simulink model "motorStyrning"  (R2020b)
settings: Solver=VariableStepAuto  StartTime=0.0  StopTime=0.1  RelTol=1e-3
model workspace (MAT data in the model file):
  intervall = 300
  intervall2 = 1
  intervall3 = 1
  timeTTT : Simulink.Signal (value not decoded)
libraries: fl_lib x116, ee_lib x24, nesl_utility x23
(part 2 of 2)

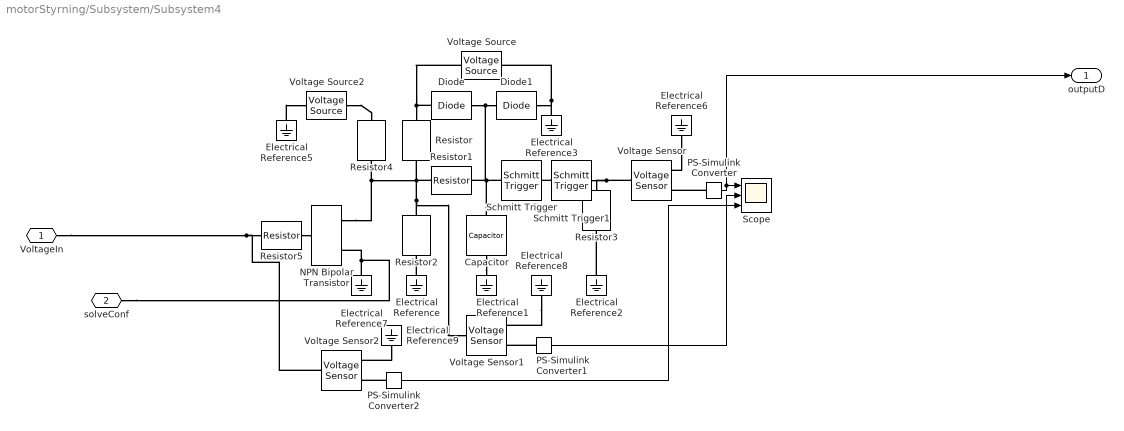
== system motorStyrning/Subsystem/Subsystem4 ==
  Capacitor : fl_lib/Electrical/Electrical Elements/Capacitor  c=100 nF  r=1e-6 Ohm  g=0 1/Ohm  i_specify=off  i_priority=None  i=0 A  i_nominal_specify=off  i_nominal_unit=A  i_nominal_value=1  v_specify=off  v_priority=None  v=0 V  v_nominal_specify=off  v_nominal_unit=V  v_nominal_value=1  vc_specify=off  vc_priority=High  vc=0 V  vc_nominal_specify=off  vc_nominal_unit=V  vc_nominal_value=1
  Diode : ee_lib/Semiconductors & Converters/Diode  ModelType=ee.enum.diode.modelType.pwl  IfMat=[.07, .12, .19, 1.75, 4.24, 7.32, 11.2; .16, .3, .72, 2.14, 4.02, 6.35, 9.12] A  TjVec=[25, 125] degC  VfVec=[.5, .7, .9, 1.3, 1.7, 2.1, 2.5] V  Vf=0.6 V  Ron=0.3 Ohm  Goff=1e-8 S  prmExp=ee.enum.diode.expParam.useTwo  I12=[.0137, .545] A  V12=[.6, .7] V  IS=1e-12 A  ec=1  I1=0.0137 A  V1=0.6 V  RS=0 Ohm  Tmeas=25 degC  N_series=1  N_parallel=1  Rz=0.3 Ohm  BV=inf V  C_param=ee.enum.diode.capParam.fixed  CJ=5 pF  CJ0=5 pF  VJ=1 V  Mgrad=0.5  Vvec=[.1, 10, 100] V  Cvec=[3.5, 1, .4] pF  FC=0.5  Q_param=ee.enum.diode.recoveryParam.off  iRM=-7.15 A  iF=4 A  didt=-750 A/us  trr_factor=3  trr=115 ns  Qrr=1500 s*uA  TT=50 ns  tau=100 ns  T_param=ee.enum.diode.temperatureParam.off  IS_T2=1.25e-7 A  I1_T2=0.245 A  V1_T2=0.5 V  Tmeas2=125 degC  EG_param=ee.enum.diode.egapParam.material_si  EG=1.11 eV  XTI_param=ee.enum.diode.xtiParam.pn  XTI=3  dBVdT=0 V/K  Tdevice=25 degC  i_specify=off  i_priority=None  i=0 A  i_nominal_specify=off  i_nominal_unit=A  i_nominal_value=1  v_specify=off  v_priority=None  v=0 V  v_nominal_specify=off  v_nominal_unit=V  v_nominal_value=1  i_capacitor_specify=off  i_capacitor_priority=None  i_capacitor=0 A  i_capacitor_nominal_specify=off  i_capacitor_nominal_unit=A  i_capacitor_nominal_value=1  v_capacitor_specify=off  v_capacitor_priority=None  v_capacitor=0 V  v_capacitor_nominal_specify=off  v_capacitor_nominal_unit=V  v_capacitor_nominal_value=1  power_dissipated_specify=off  power_dissipated_priority=None  power_dissipated=0 W  power_dissipated_nominal_specify=off  power_dissipated_nominal_unit=W  power_dissipated_nominal_value=1  thermal_network_parameterization=ee.enum.thermalNetworkTopology.cauer  Rth=[0, 10] K/W  Rth_Foster=[4, 6] K/W  thermal_mass_parameterization=ee.enum.thermalNetwork.timeconstant  thermal_mass=[0, 1] J/K  thermal_mass_Foster=[1.5, 3] J/K  thermal_time_constant=[0, 10] s  thermal_time_constant_Foster=[6, 18] s  thermal_mass_initial_temperatures=[25, 25] degC
  Diode1 : ee_lib/Semiconductors & Converters/Diode  ModelType=ee.enum.diode.modelType.pwl  IfMat=[.07, .12, .19, 1.75, 4.24, 7.32, 11.2; .16, .3, .72, 2.14, 4.02, 6.35, 9.12] A  TjVec=[25, 125] degC  VfVec=[.5, .7, .9, 1.3, 1.7, 2.1, 2.5] V  Vf=0.6 V  Ron=0.3 Ohm  Goff=1e-8 S  prmExp=ee.enum.diode.expParam.useTwo  I12=[.0137, .545] A  V12=[.6, .7] V  IS=1e-12 A  ec=1  I1=0.0137 A  V1=0.6 V  RS=0 Ohm  Tmeas=25 degC  N_series=1  N_parallel=1  Rz=0.3 Ohm  BV=inf V  C_param=ee.enum.diode.capParam.fixed  CJ=5 pF  CJ0=5 pF  VJ=1 V  Mgrad=0.5  Vvec=[.1, 10, 100] V  Cvec=[3.5, 1, .4] pF  FC=0.5  Q_param=ee.enum.diode.recoveryParam.off  iRM=-7.15 A  iF=4 A  didt=-750 A/us  trr_factor=3  trr=115 ns  Qrr=1500 s*uA  TT=50 ns  tau=100 ns  T_param=ee.enum.diode.temperatureParam.off  IS_T2=1.25e-7 A  I1_T2=0.245 A  V1_T2=0.5 V  Tmeas2=125 degC  EG_param=ee.enum.diode.egapParam.material_si  EG=1.11 eV  XTI_param=ee.enum.diode.xtiParam.pn  XTI=3  dBVdT=0 V/K  Tdevice=25 degC  i_specify=off  i_priority=None  i=0 A  i_nominal_specify=off  i_nominal_unit=A  i_nominal_value=1  v_specify=off  v_priority=None  v=0 V  v_nominal_specify=off  v_nominal_unit=V  v_nominal_value=1  i_capacitor_specify=off  i_capacitor_priority=None  i_capacitor=0 A  i_capacitor_nominal_specify=off  i_capacitor_nominal_unit=A  i_capacitor_nominal_value=1  v_capacitor_specify=off  v_capacitor_priority=None  v_capacitor=0 V  v_capacitor_nominal_specify=off  v_capacitor_nominal_unit=V  v_capacitor_nominal_value=1  power_dissipated_specify=off  power_dissipated_priority=None  power_dissipated=0 W  power_dissipated_nominal_specify=off  power_dissipated_nominal_unit=W  power_dissipated_nominal_value=1  thermal_network_parameterization=ee.enum.thermalNetworkTopology.cauer  Rth=[0, 10] K/W  Rth_Foster=[4, 6] K/W  thermal_mass_parameterization=ee.enum.thermalNetwork.timeconstant  thermal_mass=[0, 1] J/K  thermal_mass_Foster=[1.5, 3] J/K  thermal_time_constant=[0, 10] s  thermal_time_constant_Foster=[6, 18] s  thermal_mass_initial_temperatures=[25, 25] degC
  Electrical Reference{,1..3,5..9} (9 alike) : fl_lib/Electrical/Electrical Elements/Electrical Reference
  NPN Bipolar Transistor : ee_lib/Semiconductors & Converters/NPN Bipolar Transistor  parameterization=1  prmDatasheet=1  prmEquCoeff=1  BF=100  IS=1e-14 A  VAF=200 V  hfe=100  hoe=50e-6 1/Ohm  Ic_h=1 mA  Vce_h=5 V  V1=0.55 V  I1=0.5 mA  BR=1  Tmeas=25 degC  RC=0.01 Ohm  RE=1e-4 Ohm  RB=1 Ohm  C_BC=5 pF  C_BE=5 pF  TF=0 us  TR=0 us  hfe_T2=125  XTB=0  V1_T2=0.45 V  I1_T2=0.5 mA  Tmeas2=125 degC  EG=1.11 eV  XTI=3  ec=1  TdeviceDatasheet=25 degC  TdeviceEquCoeff=25 degC  thermal_network_parameterization=ee.enum.thermalNetworkTopology.cauer  Rth=[0, 10] K/W  Rth_Foster=[4, 6] K/W  thermal_mass_parameterization=ee.enum.thermalNetwork.timeconstant  thermal_mass=[0, 1] J/K  thermal_mass_Foster=[1.5, 3] J/K  thermal_time_constant=[0, 10] s  thermal_time_constant_Foster=[6, 18] s  thermal_mass_initial_temperatures=[25, 25] degC
  PS-Simulink Converter : nesl_utility/PS-Simulink Converter  PhysicalDomain=network_engine_domain  SubClassName=ps_output  LeftPortType=input  RightPortType=output  PseudoPeriodic=off  Frequencies=[]  Unit=inherit  AffineConversion=off
  PS-Simulink Converter1 : nesl_utility/PS-Simulink Converter  PhysicalDomain=network_engine_domain  SubClassName=ps_output  LeftPortType=input  RightPortType=output  PseudoPeriodic=off  Frequencies=[]  Unit=inherit  AffineConversion=off
  PS-Simulink Converter2 : nesl_utility/PS-Simulink Converter  PhysicalDomain=network_engine_domain  SubClassName=ps_output  LeftPortType=input  RightPortType=output  PseudoPeriodic=off  Frequencies=[]  Unit=inherit  AffineConversion=off
  Resistor : fl_lib/Electrical/Electrical Elements/Resistor  R=1 kOhm  i_specify=off  i_priority=None  i=0 A  i_nominal_specify=off  i_nominal_unit=A  i_nominal_value=1  v_specify=off  v_priority=None  v=0 V  v_nominal_specify=off  v_nominal_unit=V  v_nominal_value=1
  Resistor1 : fl_lib/Electrical/Electrical Elements/Resistor  R=1 kOhm  i_specify=off  i_priority=None  i=0 A  i_nominal_specify=off  i_nominal_unit=A  i_nominal_value=1  v_specify=off  v_priority=None  v=0 V  v_nominal_specify=off  v_nominal_unit=V  v_nominal_value=1
  Resistor2 : fl_lib/Electrical/Electrical Elements/Resistor  R=50 kOhm  i_specify=off  i_priority=None  i=0 A  i_nominal_specify=off  i_nominal_unit=A  i_nominal_value=1  v_specify=off  v_priority=None  v=0 V  v_nominal_specify=off  v_nominal_unit=V  v_nominal_value=1
  Resistor3 : fl_lib/Electrical/Electrical Elements/Resistor  R=10 kOhm  i_specify=off  i_priority=None  i=0 A  i_nominal_specify=off  i_nominal_unit=A  i_nominal_value=1  v_specify=off  v_priority=None  v=0 V  v_nominal_specify=off  v_nominal_unit=V  v_nominal_value=1
  Resistor4 : fl_lib/Electrical/Electrical Elements/Resistor  R=10 kOhm  i_specify=off  i_priority=None  i=0 A  i_nominal_specify=off  i_nominal_unit=A  i_nominal_value=1  v_specify=off  v_priority=None  v=0 V  v_nominal_specify=off  v_nominal_unit=V  v_nominal_value=1
  Resistor5 : fl_lib/Electrical/Electrical Elements/Resistor  R=1 kOhm  i_specify=off  i_priority=None  i=0 A  i_nominal_specify=off  i_nominal_unit=A  i_nominal_value=1  v_specify=off  v_priority=None  v=0 V  v_nominal_specify=off  v_nominal_unit=V  v_nominal_value=1
  Schmitt Trigger : ee_lib/Integrated Circuits/Logic/Schmitt Trigger  V_IL=2 V  V_IH=3 V  C_IN=5 pF  output_type=1  V_OL=0 V  V_OH=5 V  V_CC=5 V  V_meas=5 V  R_OUT=25 Ohm  R_OH=[25, 250] Ohm  I_OH=63 mA  R_OL=[30, 800] Ohm  I_OL=-45 mA  Delay=25 ns  Ron=5 Ohm  Vf=0.6 V  output_state=1
      settings: SourceProductBaseCode=PS  InternalSimscapePortConfiguration="{\"Bottom\":[],\"Left\":[{\"id\":\"A\",\"label\":\"\",\"type\":\"foundation.electrical.electrical\"}],\"Right\":[{\"id\":\"J\",\"label\":\"\",\"type\":\"foundation.electrical.electrical\"}],\"Top\":[]}"
  Schmitt Trigger1 : ee_lib/Integrated Circuits/Logic/Schmitt Trigger  V_IL=2 V  V_IH=3 V  C_IN=5 pF  output_type=1  V_OL=0 V  V_OH=5 V  V_CC=5 V  V_meas=5 V  R_OUT=25 Ohm  R_OH=[25, 250] Ohm  I_OH=63 mA  R_OL=[30, 800] Ohm  I_OL=-45 mA  Delay=25 ns  Ron=5 Ohm  Vf=0.6 V  output_state=1
      settings: SourceProductBaseCode=PS  InternalSimscapePortConfiguration="{\"Bottom\":[],\"Left\":[{\"id\":\"A\",\"label\":\"\",\"type\":\"foundation.electrical.electrical\"}],\"Right\":[{\"id\":\"J\",\"label\":\"\",\"type\":\"foundation.electrical.electrical\"}],\"Top\":[]}"
  Scope : Scope  NumInputPorts=3
  Voltage Sensor : fl_lib/Electrical/Electrical Sensors/Voltage Sensor
  Voltage Sensor1 : fl_lib/Electrical/Electrical Sensors/Voltage Sensor
  Voltage Sensor2 : fl_lib/Electrical/Electrical Sensors/Voltage Sensor
  Voltage Source : ee_lib/Sources/Voltage Source  dc_voltage=5 V  ac_voltage=0 V  ac_shift=0 rad  ac_frequency=60 Hz  noise_mode=0  PSD=0 V^2/Hz  repeatability=1  auto_seed=4112460543  user_seed=0  sample_time=1e-3 s  i_specify=off  i_priority=None  i=0 A  i_nominal_specify=off  i_nominal_unit=A  i_nominal_value=1  v_specify=off  v_priority=None  v=0 V  v_nominal_specify=off  v_nominal_unit=V  v_nominal_value=1
  Voltage Source2 : ee_lib/Sources/Voltage Source  dc_voltage=0 V  ac_voltage=0 V  ac_shift=0 rad  ac_frequency=60 Hz  noise_mode=1  PSD=0 V^2/Hz  repeatability=1  auto_seed=4144164703  user_seed=0  sample_time=1e-3 s  i_specify=off  i_priority=None  i=0 A  i_nominal_specify=off  i_nominal_unit=A  i_nominal_value=1  v_specify=off  v_priority=None  v=0 V  v_nominal_specify=off  v_nominal_unit=V  v_nominal_value=1
  VoltageIn : PMIOPort  Side=Left
  solveConf : PMIOPort  Port=2  Side=Left
  outputD : Outport
  wires:
  PS-Simulink Converter1/1 -> Scope/2
  PS-Simulink Converter2/1 -> Scope/3
  PS-Simulink Converter/1 -> outputD/1, Scope/1
  connections:
  Electrical Reference8/LConn1 -- Voltage Sensor1/RConn2
  Electrical Reference7/LConn1 -- solveConf/RConn1 -- NPN Bipolar Transistor/RConn2
  Resistor1/LConn1 -- NPN Bipolar Transistor/RConn1 -- Resistor4/RConn1 -- Resistor/RConn1 -- Resistor2/LConn1 -- Voltage Sensor1/LConn1
  Electrical Reference6/LConn1 -- Voltage Sensor/RConn2
  PS-Simulink Converter1/LConn1 -- Voltage Sensor1/RConn1
  Electrical Reference9/LConn1 -- Voltage Sensor2/RConn2
  Diode/LConn1 -- Diode1/RConn1 -- Capacitor/LConn1 -- Schmitt Trigger/LConn1 -- Resistor1/RConn1
  Voltage Source/LConn1 -- Resistor/LConn1 -- Diode/RConn1
  Electrical Reference3/LConn1 -- Voltage Source/RConn1 -- Diode1/LConn1
  PS-Simulink Converter2/LConn1 -- Voltage Sensor2/RConn1
  Electrical Reference2/LConn1 -- Resistor3/RConn1
  PS-Simulink Converter/LConn1 -- Voltage Sensor/RConn1
  Voltage Source2/LConn1 -- Resistor4/LConn1
  Voltage Sensor/LConn1 -- Resistor3/LConn1 -- Schmitt Trigger1/RConn1
  Schmitt Trigger1/LConn1 -- Schmitt Trigger/RConn1
  Voltage Sensor2/LConn1 -- Resistor5/LConn1 -- VoltageIn/RConn1
  Resistor5/RConn1 -- NPN Bipolar Transistor/LConn1
  Capacitor/RConn1 -- Electrical Reference1/LConn1
  Electrical Reference/LConn1 -- Resistor2/RConn1
  Electrical Reference5/LConn1 -- Voltage Source2/RConn1

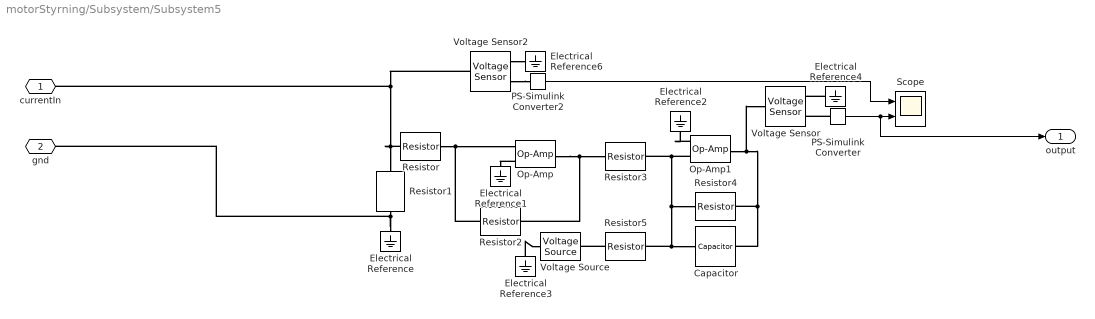
== system motorStyrning/Subsystem/Subsystem5 ==
  Capacitor : fl_lib/Electrical/Electrical Elements/Capacitor  c=10 nF  r=1e-6 Ohm  g=0 1/Ohm  i_specify=off  i_priority=None  i=0 A  i_nominal_specify=off  i_nominal_unit=A  i_nominal_value=1  v_specify=off  v_priority=None  v=0 V  v_nominal_specify=off  v_nominal_unit=V  v_nominal_value=1  vc_specify=off  vc_priority=High  vc=0 V  vc_nominal_specify=off  vc_nominal_unit=V  vc_nominal_value=1
  Electrical Reference{,1..4,6} (6 alike) : fl_lib/Electrical/Electrical Elements/Electrical Reference
  Op-Amp : fl_lib/Electrical/Electrical Elements/Op-Amp  outI_specify=off  outI_priority=None  outI=0 A  outI_nominal_specify=off  outI_nominal_unit=A  outI_nominal_value=1
  Op-Amp1 : fl_lib/Electrical/Electrical Elements/Op-Amp  outI_specify=off  outI_priority=None  outI=0 A  outI_nominal_specify=off  outI_nominal_unit=A  outI_nominal_value=1
  PS-Simulink Converter : nesl_utility/PS-Simulink Converter  PhysicalDomain=network_engine_domain  SubClassName=ps_output  LeftPortType=input  RightPortType=output  PseudoPeriodic=off  Frequencies=[]  Unit=inherit  AffineConversion=off
  PS-Simulink Converter2 : nesl_utility/PS-Simulink Converter  PhysicalDomain=network_engine_domain  SubClassName=ps_output  LeftPortType=input  RightPortType=output  PseudoPeriodic=off  Frequencies=[]  Unit=inherit  AffineConversion=off
  Resistor : fl_lib/Electrical/Electrical Elements/Resistor  R=10 kOhm  i_specify=off  i_priority=None  i=0 A  i_nominal_specify=off  i_nominal_unit=A  i_nominal_value=1  v_specify=off  v_priority=None  v=0 V  v_nominal_specify=off  v_nominal_unit=V  v_nominal_value=1
  Resistor1 : fl_lib/Electrical/Electrical Elements/Resistor  R=60 Ohm  i_specify=off  i_priority=None  i=0 A  i_nominal_specify=off  i_nominal_unit=A  i_nominal_value=1  v_specify=off  v_priority=None  v=0 V  v_nominal_specify=off  v_nominal_unit=V  v_nominal_value=1
  Resistor2 : fl_lib/Electrical/Electrical Elements/Resistor  R=8275 Ohm  i_specify=off  i_priority=None  i=0 A  i_nominal_specify=off  i_nominal_unit=A  i_nominal_value=1  v_specify=off  v_priority=None  v=0 V  v_nominal_specify=off  v_nominal_unit=V  v_nominal_value=1
  Resistor3 : fl_lib/Electrical/Electrical Elements/Resistor  R=10 kOhm  i_specify=off  i_priority=None  i=0 A  i_nominal_specify=off  i_nominal_unit=A  i_nominal_value=1  v_specify=off  v_priority=None  v=0 V  v_nominal_specify=off  v_nominal_unit=V  v_nominal_value=1
  Resistor4 : fl_lib/Electrical/Electrical Elements/Resistor  R=10 kOhm  i_specify=off  i_priority=None  i=0 A  i_nominal_specify=off  i_nominal_unit=A  i_nominal_value=1  v_specify=off  v_priority=None  v=0 V  v_nominal_specify=off  v_nominal_unit=V  v_nominal_value=1
  Resistor5 : fl_lib/Electrical/Electrical Elements/Resistor  R=29.7 kOhm  i_specify=off  i_priority=None  i=0 A  i_nominal_specify=off  i_nominal_unit=A  i_nominal_value=1  v_specify=off  v_priority=None  v=0 V  v_nominal_specify=off  v_nominal_unit=V  v_nominal_value=1
  Scope : Scope  NumInputPorts=2
  Voltage Sensor : fl_lib/Electrical/Electrical Sensors/Voltage Sensor
  Voltage Sensor2 : fl_lib/Electrical/Electrical Sensors/Voltage Sensor
  Voltage Source : ee_lib/Sources/Voltage Source  dc_voltage=-15 V  ac_voltage=0 V  ac_shift=0 rad  ac_frequency=60 Hz  noise_mode=0  PSD=0 V^2/Hz  repeatability=1  auto_seed=3243031446  user_seed=0  sample_time=1e-3 s  i_specify=off  i_priority=None  i=0 A  i_nominal_specify=off  i_nominal_unit=A  i_nominal_value=1  v_specify=off  v_priority=None  v=0 V  v_nominal_specify=off  v_nominal_unit=V  v_nominal_value=1
  currentIn : PMIOPort  Side=Left
  gnd : PMIOPort  Port=2  Side=Left
  output : Outport
  wires:
  PS-Simulink Converter/1 -> output/1, Scope/2
  PS-Simulink Converter2/1 -> Scope/1
  connections:
  Resistor1/RConn1 -- gnd/RConn1 -- Electrical Reference/LConn1
  Voltage Sensor2/RConn1 -- PS-Simulink Converter2/LConn1
  Voltage Sensor2/RConn2 -- Electrical Reference6/LConn1
  PS-Simulink Converter/LConn1 -- Voltage Sensor/RConn1
  Resistor5/LConn1 -- Voltage Source/LConn1
  Op-Amp/LConn2 -- Electrical Reference1/LConn1
  Op-Amp1/LConn2 -- Resistor3/RConn1 -- Resistor5/RConn1 -- Capacitor/LConn1 -- Resistor4/LConn1
  Electrical Reference3/LConn1 -- Voltage Source/RConn1
  Electrical Reference4/LConn1 -- Voltage Sensor/RConn2
  Op-Amp1/LConn1 -- Electrical Reference2/LConn1
  Capacitor/RConn1 -- Resistor4/RConn1 -- Op-Amp1/RConn1 -- Voltage Sensor/LConn1
  Op-Amp/RConn1 -- Resistor3/LConn1 -- Resistor2/RConn1
  Resistor/RConn1 -- Resistor2/LConn1 -- Op-Amp/LConn1
  Voltage Sensor2/LConn1 -- Resistor/LConn1 -- Resistor1/LConn1 -- currentIn/RConn1

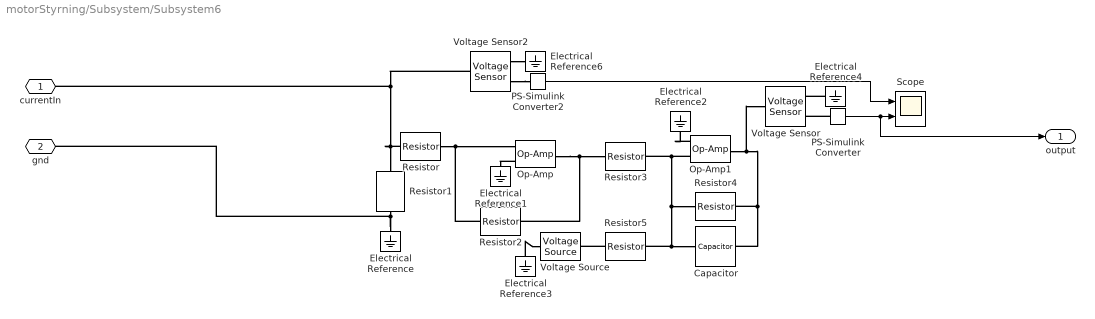
== system motorStyrning/Subsystem/Subsystem6 ==
  Capacitor : fl_lib/Electrical/Electrical Elements/Capacitor  c=10 nF  r=1e-6 Ohm  g=0 1/Ohm  i_specify=off  i_priority=None  i=0 A  i_nominal_specify=off  i_nominal_unit=A  i_nominal_value=1  v_specify=off  v_priority=None  v=0 V  v_nominal_specify=off  v_nominal_unit=V  v_nominal_value=1  vc_specify=off  vc_priority=High  vc=0 V  vc_nominal_specify=off  vc_nominal_unit=V  vc_nominal_value=1
  Electrical Reference{,1..4,6} (6 alike) : fl_lib/Electrical/Electrical Elements/Electrical Reference
  Op-Amp : fl_lib/Electrical/Electrical Elements/Op-Amp  outI_specify=off  outI_priority=None  outI=0 A  outI_nominal_specify=off  outI_nominal_unit=A  outI_nominal_value=1
  Op-Amp1 : fl_lib/Electrical/Electrical Elements/Op-Amp  outI_specify=off  outI_priority=None  outI=0 A  outI_nominal_specify=off  outI_nominal_unit=A  outI_nominal_value=1
  PS-Simulink Converter : nesl_utility/PS-Simulink Converter  PhysicalDomain=network_engine_domain  SubClassName=ps_output  LeftPortType=input  RightPortType=output  PseudoPeriodic=off  Frequencies=[]  Unit=inherit  AffineConversion=off
  PS-Simulink Converter2 : nesl_utility/PS-Simulink Converter  PhysicalDomain=network_engine_domain  SubClassName=ps_output  LeftPortType=input  RightPortType=output  PseudoPeriodic=off  Frequencies=[]  Unit=inherit  AffineConversion=off
  Resistor : fl_lib/Electrical/Electrical Elements/Resistor  R=10 kOhm  i_specify=off  i_priority=None  i=0 A  i_nominal_specify=off  i_nominal_unit=A  i_nominal_value=1  v_specify=off  v_priority=None  v=0 V  v_nominal_specify=off  v_nominal_unit=V  v_nominal_value=1
  Resistor1 : fl_lib/Electrical/Electrical Elements/Resistor  R=60 Ohm  i_specify=off  i_priority=None  i=0 A  i_nominal_specify=off  i_nominal_unit=A  i_nominal_value=1  v_specify=off  v_priority=None  v=0 V  v_nominal_specify=off  v_nominal_unit=V  v_nominal_value=1
  Resistor2 : fl_lib/Electrical/Electrical Elements/Resistor  R=8275 Ohm  i_specify=off  i_priority=None  i=0 A  i_nominal_specify=off  i_nominal_unit=A  i_nominal_value=1  v_specify=off  v_priority=None  v=0 V  v_nominal_specify=off  v_nominal_unit=V  v_nominal_value=1
  Resistor3 : fl_lib/Electrical/Electrical Elements/Resistor  R=10 kOhm  i_specify=off  i_priority=None  i=0 A  i_nominal_specify=off  i_nominal_unit=A  i_nominal_value=1  v_specify=off  v_priority=None  v=0 V  v_nominal_specify=off  v_nominal_unit=V  v_nominal_value=1
  Resistor4 : fl_lib/Electrical/Electrical Elements/Resistor  R=10 kOhm  i_specify=off  i_priority=None  i=0 A  i_nominal_specify=off  i_nominal_unit=A  i_nominal_value=1  v_specify=off  v_priority=None  v=0 V  v_nominal_specify=off  v_nominal_unit=V  v_nominal_value=1
  Resistor5 : fl_lib/Electrical/Electrical Elements/Resistor  R=29.7 kOhm  i_specify=off  i_priority=None  i=0 A  i_nominal_specify=off  i_nominal_unit=A  i_nominal_value=1  v_specify=off  v_priority=None  v=0 V  v_nominal_specify=off  v_nominal_unit=V  v_nominal_value=1
  Scope : Scope  NumInputPorts=2
  Voltage Sensor : fl_lib/Electrical/Electrical Sensors/Voltage Sensor
  Voltage Sensor2 : fl_lib/Electrical/Electrical Sensors/Voltage Sensor
  Voltage Source : ee_lib/Sources/Voltage Source  dc_voltage=-15 V  ac_voltage=0 V  ac_shift=0 rad  ac_frequency=60 Hz  noise_mode=0  PSD=0 V^2/Hz  repeatability=1  auto_seed=4112460543  user_seed=0  sample_time=1e-3 s  i_specify=off  i_priority=None  i=0 A  i_nominal_specify=off  i_nominal_unit=A  i_nominal_value=1  v_specify=off  v_priority=None  v=0 V  v_nominal_specify=off  v_nominal_unit=V  v_nominal_value=1
  currentIn : PMIOPort  Side=Left
  gnd : PMIOPort  Port=2  Side=Left
  output : Outport
  wires:
  PS-Simulink Converter/1 -> output/1, Scope/2
  PS-Simulink Converter2/1 -> Scope/1
  connections:
  Resistor1/RConn1 -- Electrical Reference/LConn1 -- gnd/RConn1
  Voltage Sensor2/RConn1 -- PS-Simulink Converter2/LConn1
  Voltage Sensor2/RConn2 -- Electrical Reference6/LConn1
  PS-Simulink Converter/LConn1 -- Voltage Sensor/RConn1
  Resistor5/LConn1 -- Voltage Source/LConn1
  Op-Amp/LConn2 -- Electrical Reference1/LConn1
  Op-Amp1/LConn2 -- Resistor3/RConn1 -- Resistor5/RConn1 -- Capacitor/LConn1 -- Resistor4/LConn1
  Electrical Reference3/LConn1 -- Voltage Source/RConn1
  Electrical Reference4/LConn1 -- Voltage Sensor/RConn2
  Op-Amp1/LConn1 -- Electrical Reference2/LConn1
  Capacitor/RConn1 -- Resistor4/RConn1 -- Op-Amp1/RConn1 -- Voltage Sensor/LConn1
  Op-Amp/RConn1 -- Resistor3/LConn1 -- Resistor2/RConn1
  Resistor/RConn1 -- Resistor2/LConn1 -- Op-Amp/LConn1
  Voltage Sensor2/LConn1 -- Resistor/LConn1 -- Resistor1/LConn1 -- currentIn/RConn1

== matlab function motorStyrning/Subsystem/MATLAB Function ==
  data: freeW input; u input; y output
function y = fcn(freeW, u)
%#codegen
if u == 2
    
    if freeW==0
    a0 = 0; a1 = 0; a2 = 10; b0 = 10; b1 = 0; b2 = 10;  %% a2 var 10 innan AW ändrade
    else
    a0 = 0; a1 = 0; a2 = 10; b0 = 0; b1 = 0; b2 = 10;   %% a2 var 10 innan AW ändrade
    end
    
elseif u == 10 || 32
    
    if freeW == 0
      a0 = 0; a1 = 10; a2 = 0; b0 = 10; b1 = 10; b2 = 0;  
    else
        a0 = 0; a1 = 10; a2 = 0; b0 = 0; b1 = 10; b2 = 0;
    end
elseif u == 20
        
    if freeW == 0
        a0 = 10; a1 = 0; a2 = 0; b0 = 10; b1 = 0; b2 = 10;
    else
       a0 = 10; a1 = 0; a2 = 0; b0 = 10; b1 = 0; b2 = 0; 
    end
elseif u == 12
        
    if freeW == 0
        a0 = 0; a1 = 0; a2 = 10; b0 = 10; b1 = 0; b2 = 10;
    else
        a0 = 0; a1 = 0; a2 = 0; b0 = 10; b1 = 0; b2 = 0;
    end
elseif u == 30
        
    if freeW == 0
        a0 = 0; a1 = 10; a2 = 0; b0 = 0; b1 = 10; b2 = 10;
    else
        a0 = 0; a1 = 0; a2 = 0; b0 = 0; b1 = 0; b2 = 10;
    end
elseif u == 22
        
    if freeW == 0
        a0 = 10; a1 = 0; a2 = 0; b0 = 10; b1 = 10; b2 = 0;
    else
        a0 = 0; a1 = 0; a2 = 0; b0 = 10; b1 = 0; b2 = 0;
    end
end

A = [a0,a1,a2,b0,b1,b2]';

y = A;

== matlab function motorStyrning/Subsystem/MATLAB Function2 ==
  data: u2 input; u1 input; u input; y output
function y = fcn(u2, u1, u)

A = [u,u1,u2]';

for n = 1 : length(A)
    A(n) = abs(A(n) * 50 - 250);
    if A(n) <= 251
         A(n) = 0;
    else
         A(n) = 1;
    end
end

if sum(A) > 0
    y = 1;
else
    y = 0;
end

== matlab function motorStyrning/Subsystem/MATLAB Function1 ==
  data: freeW input; u input; y output
function y = fcn(freeW, u)
%#codegen
%if u == 2
    %a0 = 0; a1 = 10; a2 = 10; b0 = 0; b1 = 10; b2 = 10;
%elseif u == 10 || 32
       % a0 = 0; a1 = 10; a2 = 0; b0 = 10; b1 = 10; b2 = 0;
%elseif u == 20
       % a0 = 10; a1 = 0; a2 = 0; b0 = 0; b1 = 10; b2 = 10;
%elseif u == 12
      %  a0 = 0; a1 = 00; a2 = 10; b0 = 10; b1 = 0; b2 = 10;
%elseif u == 30
      %  a0 = 0; a1 = 10; a2 = 0; b0 = 0; b1 = 10; b2 = 10;
%elseif u == 22
       % a0 = 10; a1 = 00; a2 = 0; b0 = 10; b1 = 10; b2 = 0;
%end

if u == 2
    
    if freeW==0
        t0 = 0; t1 = 0; t2 = 10; t3 = 0; t4 = 10; t5 = 0;  
    else
        t0 = 0; t1 = 0; t2 = 10; t3 = 0; t4 = 0; t5 = 0;  
    end
    
elseif u == 10 || 32
    
    if freeW == 0
         t0 = 0; t1 = 10; t2 = 0; t3 = 10; t4 = 0; t5 = 0;  
    else
         t0 = 0; t1 = 0; t2 = 0; t3 = 0; t4 = 0; t5 = 0;
    end
    
elseif u == 20
    
    if freeW == 0
        t0 = 10; t1 = 0; t2 = 0; t3 = 10; t4 = 0; t5 = 10;  
    else
        t0 = 0; t1 = 0; t2 = 0; t3 = 0; t4 = 0; t5 = 10;
    end
    
elseif u == 12
    
    if freeW == 0
        t0 = 0; t1 = 0; t2 = 10; t3 = 10; t4 = 0; t5 = 0;  
    else
        t0 = 0; t1 = 0; t2 = 10; t3 = 0; t4 = 0; t5 = 0;
    end
    
elseif u == 30
    
    if freeW == 0
        t0 = 0; t1 = 10; t2 = 0; t3 = 0; t4 = 0; t5 = 10;  
    else
        t0 = 0; t1 = 10; t2 = 0; t3 = 0; t4 = 0; t5 = 0;
    end
    
elseif u == 22
    
    if freeW == 0
        t0 = 10; t1 = 0; t2 = 0; t3 = 0; t4 = 10; t5 = 0;  
    else
        t0 = 0; t1 = 0; t2 = 0; t3 = 0; t4 = 10; t5 = 0;
    end
end
    
    
A = [t0,t1,t2,t3,t4,t5]';
%if freeW >= 1
   % for n = 1 : length(A)
    %  if sum(A) > 10
     %     A(n) = 0;
     % end
  %  end
%end
y = A;
